simulink library "LIBRARY_SAD"  (R2025b)
settings: Solver=VariableStepAuto  StartTime=0.0  StopTime=10.0  RelTol=1e-3
values from neighbouring files (symbols this model uses):
  c = astroConstants(5)*1e3    [SCRIPT_SAD_DEMO.m]
  eps_E = deg2rad(astroConstants(63))    [SCRIPT_SAD_DEMO.m]
  F0 = 237    [SCRIPT_SAD_DEMO.m]
  F_e = 1358    [SCRIPT_SAD_DEMO.m]
  g = zeros(N, N+1)    [SCRIPT_SAD_DEMO.m]
  h = zeros(N, N+1)    [SCRIPT_SAD_DEMO.m]
  j_B = [0.01; 0.05; 0.01]    [SCRIPT_SAD_DEMO.m]
  JD0 = juliandate(startTime)    [SCRIPT_SAD_DEMO.m]
  mu = astroConstants(13)    [SCRIPT_SAD_DEMO.m]
  n = sqrt( (mu/ (a)^3))    [SCRIPT_SAD_DEMO.m]
  N = 13    [SCRIPT_SAD_DEMO.m]
  n_sun = 2*pi/T_sun    (= 1.99238499086e-07)    [SCRIPT_SAD_DEMO.m]
  r_sun = 1*AU    [SCRIPT_SAD_DEMO.m]
  Re = astroConstants(23)    [SCRIPT_SAD_DEMO.m]
  SRP = SRP_nom    [SCRIPT_SAD_DEMO.m]
  t0 = 0    [SCRIPT_SAD_DEMO.m]
  theta = 0    [SCRIPT_SAD_DEMO.m]
  w0 = w0_nom    [SCRIPT_SAD_DEMO.m]
  w_E = deg2rad(15.04)/3600    [SCRIPT_SAD_DEMO.m]
undefined symbols (not defined in the file or in its folder): g0_1, g1_1, h1_1, Ix, Iy, Iz, phi0, psi0, theta0
libraries: matrix_library x13, lIBRARY_SAD_SAD x12, $bdroot x5, LIBRARY_SAD_SAD x3, simulink x1
(part 1 of 2)
settings Model: Creator=fabio  LastModifiedBy=tomasfadista

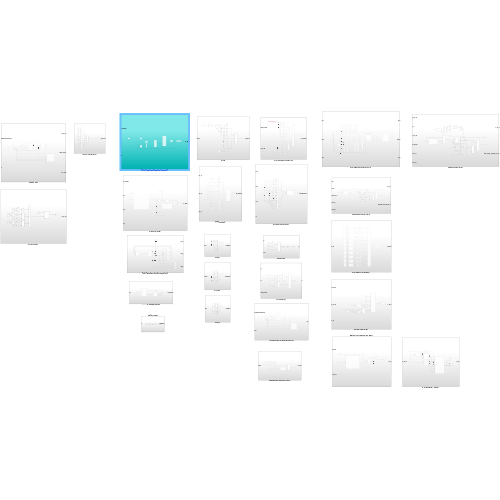
[thumbnail: Simulink's stored preview of the top-level diagram]
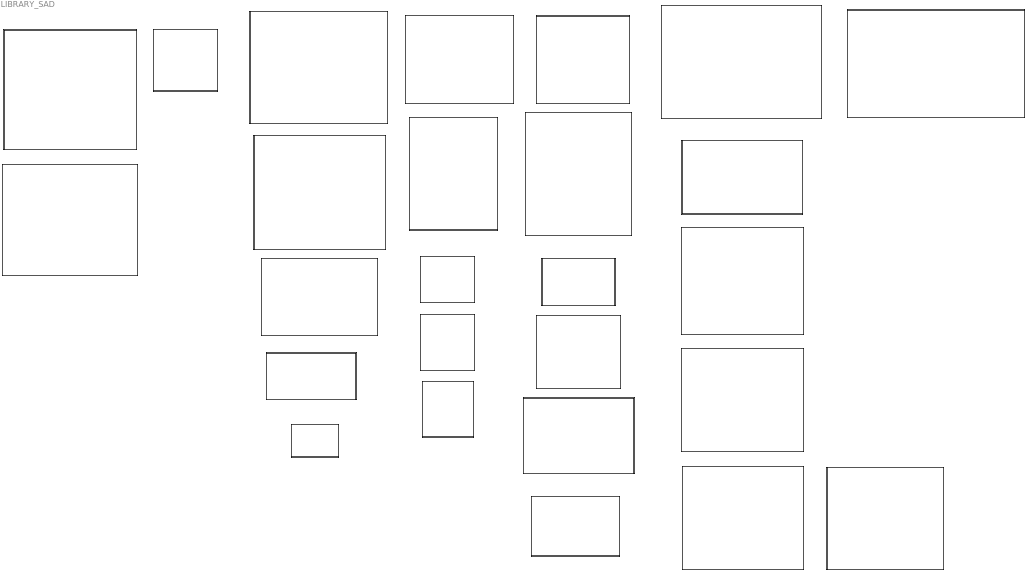
== system LIBRARY_SAD ==
  A1(theta) : Subsystem
  A2(psi) : Subsystem
  A3(phi) : Subsystem
  A_LVLH : Subsystem
  A_LVLH (elliptical,inclined orbit) : Subsystem
  B_N (IGRF Model - Order N) : Subsystem
  Conic Equation : Subsystem
  DCM Orthonormalisation : Subsystem
  DCM w matrix : Subsystem
  Earth Radiation Pressure : Subsystem
  Earth's Magnetic Dipole (unit vector) : Subsystem
  Earth-S/C Orbit : Subsystem
  Euler Angles Kinematics (seq. 312) : Subsystem
  "Euler Equations (scalar, torque-free)" : Subsystem
  Euler Equations Dynamics (vectorial) : Subsystem
  Gravity Gradient Torque : Subsystem
  I_matrix (principal axis) : Subsystem
  Kinematics (DCM) : Subsystem
  "Magnetic Torque (Simple Dipole Model) " : Subsystem
  Orbital Period : Subsystem
  Quaternion Omega matrix : Subsystem
  Solar Radiation Pressure Force : Subsystem
  Solar Radiation Torque (SRP) : Subsystem
  Sun-Earth Orbit : Subsystem
  Two-body Dynamics (keplerian elements) : Subsystem
  vector_norm : Subsystem

== system LIBRARY_SAD/A1(theta) ==
  theta : Inport
  Constant{,1,3..4} (4 alike) : Constant  Value=0
  Constant2 : Constant
  Cos : Trigonometry  Operator=cos
  Cos1 : Trigonometry  Operator=cos
  Gain : Gain  Gain=-1
  Sin : Trigonometry
  Sin1 : Trigonometry
  Vector Concatenate : Concatenate  NumInputs=3
  Vector Concatenate1 : Concatenate  NumInputs=3
  Vector Concatenate2 : Concatenate  NumInputs=3
  Vector Concatenate3 : Concatenate  NumInputs=3  Mode=Multidimensional array  ConcatenateDimension=2
  A1(theta) : Outport
  wires:
  Vector Concatenate3/1 -> A1(theta)/1
  Vector Concatenate2/1 -> Vector Concatenate3/1
  Vector Concatenate1/1 -> Vector Concatenate3/3
  Constant2/1 -> Vector Concatenate2/1
  Constant3/1 -> Vector Concatenate2/2
  Constant4/1 -> Vector Concatenate2/3
  Constant1/1 -> Vector Concatenate1/1
  Cos1/1 -> Vector Concatenate1/3
  Sin1/1 -> Vector Concatenate1/2
  Vector Concatenate/1 -> Vector Concatenate3/2
  Constant/1 -> Vector Concatenate/1
  Gain/1 -> Vector Concatenate/3
  Cos/1 -> Vector Concatenate/2
  Sin/1 -> Gain/1
  theta/1 -> Cos1/1, Sin1/1, Sin/1, Cos/1

== system LIBRARY_SAD/A2(psi) ==
  psi : Inport
  Constant{,1,3..4} (4 alike) : Constant  Value=0
  Constant2 : Constant
  Cos : Trigonometry  Operator=cos
  Cos1 : Trigonometry  Operator=cos
  Gain : Gain  Gain=-1
  Sin : Trigonometry
  Sin1 : Trigonometry
  Vector Concatenate : Concatenate  NumInputs=3
  Vector Concatenate1 : Concatenate  NumInputs=3
  Vector Concatenate2 : Concatenate  NumInputs=3
  Vector Concatenate3 : Concatenate  NumInputs=3  Mode=Multidimensional array  ConcatenateDimension=2
  A2(psi) : Outport
  wires:
  psi/1 -> Cos1/1, Sin1/1, Sin/1, Cos/1
  Vector Concatenate/1 -> Vector Concatenate3/2
  Vector Concatenate1/1 -> Vector Concatenate3/3
  Vector Concatenate2/1 -> Vector Concatenate3/1
  Vector Concatenate3/1 -> A2(psi)/1
  Cos/1 -> Vector Concatenate2/1
  Constant/1 -> Vector Concatenate2/2
  Sin/1 -> Vector Concatenate2/3
  Constant1/1 -> Vector Concatenate/1
  Constant2/1 -> Vector Concatenate/2
  Constant3/1 -> Vector Concatenate/3
  Sin1/1 -> Gain/1
  Constant4/1 -> Vector Concatenate1/2
  Cos1/1 -> Vector Concatenate1/3
  Gain/1 -> Vector Concatenate1/1

== system LIBRARY_SAD/A3(phi) ==
  phi : Inport
  Constant{,1..3} (4 alike) : Constant  Value=0
  Constant4 : Constant
  Cos : Trigonometry  Operator=cos
  Cos1 : Trigonometry  Operator=cos
  Gain : Gain  Gain=-1
  Sin : Trigonometry
  Sin1 : Trigonometry
  Vector Concatenate : Concatenate  NumInputs=3
  Vector Concatenate1 : Concatenate  NumInputs=3
  Vector Concatenate2 : Concatenate  NumInputs=3
  Vector Concatenate3 : Concatenate  NumInputs=3  Mode=Multidimensional array  ConcatenateDimension=2
  A3(phi) : Outport
  wires:
  phi/1 -> Sin1/1, Cos/1, Sin/1, Cos1/1
  Sin/1 -> Gain/1
  Cos/1 -> Vector Concatenate/1
  Gain/1 -> Vector Concatenate/2
  Constant/1 -> Vector Concatenate/3
  Vector Concatenate/1 -> Vector Concatenate3/1
  Sin1/1 -> Vector Concatenate1/1
  Cos1/1 -> Vector Concatenate1/2
  Constant1/1 -> Vector Concatenate1/3
  Constant4/1 -> Vector Concatenate2/3
  Constant3/1 -> Vector Concatenate2/2
  Constant2/1 -> Vector Concatenate2/1
  Vector Concatenate1/1 -> Vector Concatenate3/2
  Vector Concatenate2/1 -> Vector Concatenate3/3
  Vector Concatenate3/1 -> A3(phi)/1

== system LIBRARY_SAD/A_LVLH ==
  Time : Inport
  Constant : Constant  Value=0
  Constant1 : Constant
  Cos : Trigonometry  Operator=cos
  Gain1 : Gain  Gain=n
  Gain2 : Gain  Gain=-1
  Sin : Trigonometry
  Vector Concatenate : Concatenate  NumInputs=3
  Vector Concatenate1 : Concatenate  NumInputs=3
  Vector Concatenate2 : Concatenate  NumInputs=3
  Vector Concatenate3 : Concatenate  NumInputs=3  Mode=Multidimensional array  ConcatenateDimension=2
  A_LVLH : Outport
  wires:
  Constant/1 -> Vector Concatenate2/2, Vector Concatenate2/1, Vector Concatenate1/3, Vector Concatenate/3
  Gain2/1 -> Vector Concatenate/2
  Cos/1 -> Vector Concatenate1/2, Vector Concatenate/1
  Gain1/1 -> Sin/1, Cos/1
  Sin/1 -> Vector Concatenate1/1, Gain2/1
  Vector Concatenate1/1 -> Vector Concatenate3/2
  Vector Concatenate3/1 -> A_LVLH/1
  Vector Concatenate2/1 -> Vector Concatenate3/3
  Vector Concatenate/1 -> Vector Concatenate3/1
  Time/1 -> Gain1/1
  Constant1/1 -> Vector Concatenate2/3

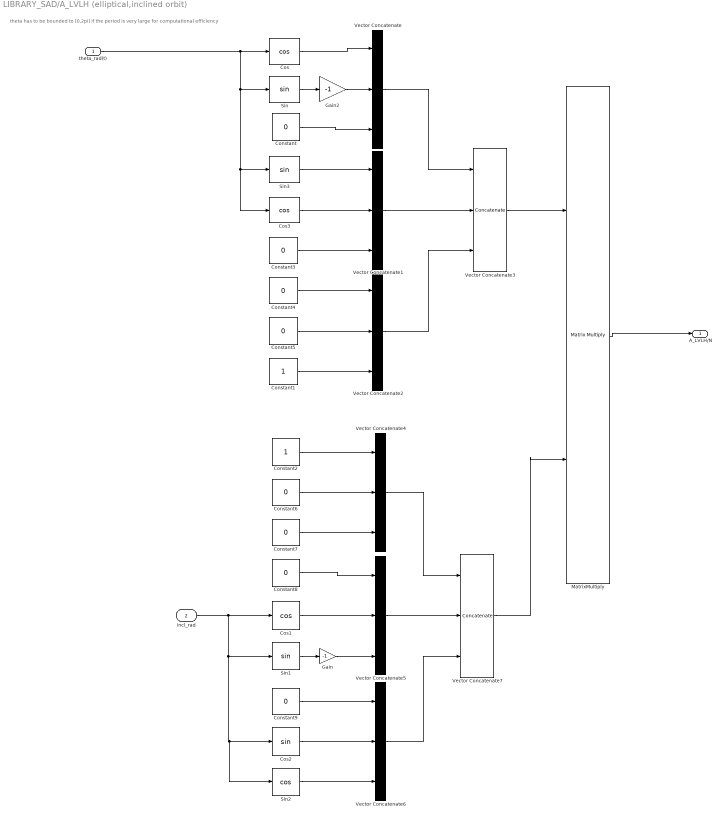
== system LIBRARY_SAD/A_LVLH (elliptical,inclined orbit) ==
  note: theta has to be bounded to [0,2pi] if the period is very large for computational efficiency
  theta_rad(t) : Inport
  incl_rad : Inport  Port=2
  Constant{,3..9} (8 alike) : Constant  Value=0
  Constant1 : Constant
  Constant2 : Constant
  Cos : Trigonometry  Operator=cos
  Cos1 : Trigonometry  Operator=cos
  Cos2 : Trigonometry
  Cos3 : Trigonometry  Operator=cos
  Gain : Gain  Gain=-1
  Gain2 : Gain  Gain=-1
  MatrixMultiply : Product  Multiplication=Matrix(*)
  Sin : Trigonometry
  Sin1 : Trigonometry
  Sin2 : Trigonometry  Operator=cos
  Sin3 : Trigonometry
  Vector Concatenate{,1..2,4..6} (6 alike) : Concatenate  NumInputs=3
  Vector Concatenate3 : Concatenate  NumInputs=3  Mode=Multidimensional array  ConcatenateDimension=2
  Vector Concatenate7 : Concatenate  NumInputs=3  Mode=Multidimensional array  ConcatenateDimension=2
  A_LVLH/N : Outport
  wires:
  Constant/1 -> Vector Concatenate/3
  Gain2/1 -> Vector Concatenate/2
  Cos/1 -> Vector Concatenate/1
  theta_rad(t)/1 -> Cos3/1, Sin3/1, Sin/1, Cos/1
  Sin/1 -> Gain2/1
  Vector Concatenate1/1 -> Vector Concatenate3/2
  Vector Concatenate3/1 -> MatrixMultiply/1
  Vector Concatenate2/1 -> Vector Concatenate3/3
  Vector Concatenate/1 -> Vector Concatenate3/1
  Constant1/1 -> Vector Concatenate2/3
  MatrixMultiply/1 -> A_LVLH/N/1
  Constant2/1 -> Vector Concatenate4/1
  incl_rad/1 -> Sin2/1, Cos2/1, Sin1/1, Cos1/1
  Cos1/1 -> Vector Concatenate5/2
  Sin1/1 -> Gain/1
  Gain/1 -> Vector Concatenate5/3
  Cos2/1 -> Vector Concatenate6/2
  Sin2/1 -> Vector Concatenate6/3
  Vector Concatenate5/1 -> Vector Concatenate7/2
  Vector Concatenate4/1 -> Vector Concatenate7/1
  Vector Concatenate6/1 -> Vector Concatenate7/3
  Vector Concatenate7/1 -> MatrixMultiply/2
  Sin3/1 -> Vector Concatenate1/1
  Cos3/1 -> Vector Concatenate1/2
  Constant3/1 -> Vector Concatenate1/3
  Constant4/1 -> Vector Concatenate2/1
  Constant5/1 -> Vector Concatenate2/2
  Constant6/1 -> Vector Concatenate4/2
  Constant7/1 -> Vector Concatenate4/3
  Constant8/1 -> Vector Concatenate5/1
  Constant9/1 -> Vector Concatenate6/1

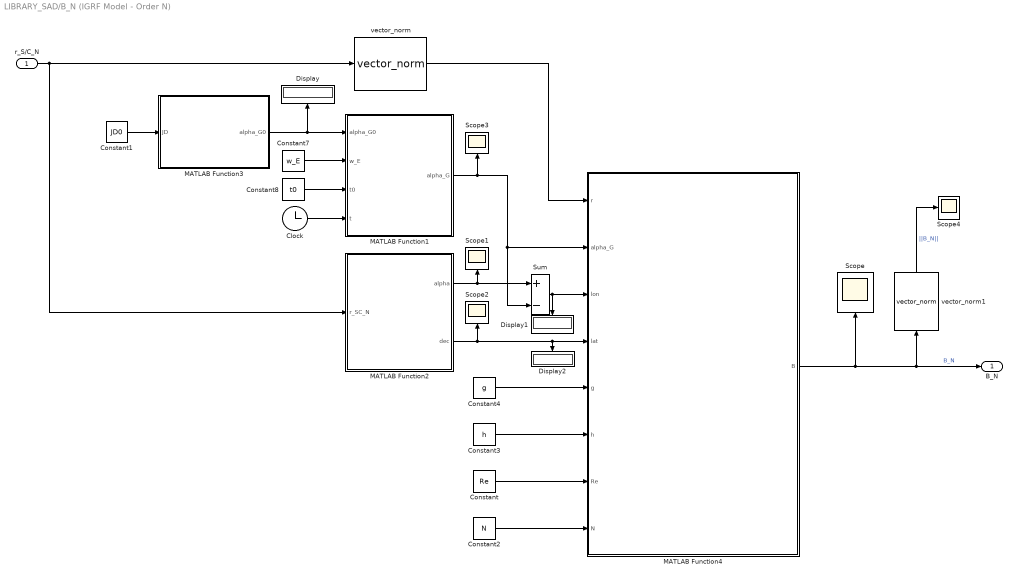
== system LIBRARY_SAD/B_N (IGRF Model - Order N) ==
  r_S/C_N : Inport
  Clock : Clock
  Constant : Constant  Value=Re
  Constant1 : Constant  Value=JD0
  Constant2 : Constant  Value=N
  Constant3 : Constant  Value=h
  Constant4 : Constant  Value=g
  Constant7 : Constant  Value=w_E
  Constant8 : Constant  Value=t0
  Display : Display
  Display1 : Display
  Display2 : Display
  MATLAB Function1 : MATLAB Function  TreatAsAtomicUnit=on
  MATLAB Function2 : MATLAB Function  TreatAsAtomicUnit=on
  MATLAB Function3 : MATLAB Function  TreatAsAtomicUnit=on
  MATLAB Function4 : MATLAB Function  TreatAsAtomicUnit=on
  Scope{,1..4} (5 alike) : Scope
      Scope settings: ActiveDisplayYMinimum=-1.512041376614329E-5  ActiveDisplayYMaximum=2.8400469726666671E-5  DataLoggingVariableName=ScopeData27
      Scope1 settings: ActiveDisplayYMinimum=-1  ActiveDisplayYMaximum=1  DataLoggingVariableName=ScopeData28
      Scope2 settings: ActiveDisplayYMinimum=-1  ActiveDisplayYMaximum=1  DataLoggingVariableName=ScopeData29
      Scope3 settings: ActiveDisplayYMinimum=-1  ActiveDisplayYMaximum=1  DataLoggingVariableName=ScopeData30
      Scope4 settings: ActiveDisplayYMinimum=-1  ActiveDisplayYMaximum=1  DataLoggingVariableName=ScopeData32
  Sum : Sum  Inputs=+-
  vector_norm : $bdroot/vector_norm  SystemSampleTime=-1  VariantActivationTime=update diagram  EmptyChoice=off  PassThrough=off  PassThroughVariantControl=(default)  EmptyChoiceVariantControl=(default)  AllowFlexibleInterface=on  Latency=0  AutoFrameSizeCalculation=off
  vector_norm1 : $bdroot/vector_norm  SystemSampleTime=-1  VariantActivationTime=update diagram  EmptyChoice=off  PassThrough=off  PassThroughVariantControl=(default)  EmptyChoiceVariantControl=(default)  AllowFlexibleInterface=on  Latency=0  AutoFrameSizeCalculation=off
  B_N : Outport
  wires:
  Constant1/1 -> MATLAB Function3/1(JD)
  MATLAB Function2/1(alpha) -> Sum/1, Scope1/1
  Sum/1 -> Display1/1, MATLAB Function4/3(lon)
  MATLAB Function2/2(dec) -> Display2/1, MATLAB Function4/4(lat), Scope2/1
  MATLAB Function1/1(alpha_G) -> Scope3/1, Sum/2, MATLAB Function4/2(alpha_G)
  Clock/1 -> MATLAB Function1/4(t)
  Constant8/1 -> MATLAB Function1/3(t0)
  Constant7/1 -> MATLAB Function1/2(w_E)
  vector_norm1/1 -> Scope4/1  "||B_N||"
  MATLAB Function4/1(B) -> Scope/1, vector_norm1/1, B_N/1  "B_N"
  Constant4/1 -> MATLAB Function4/5(g)
  Constant3/1 -> MATLAB Function4/6(h)
  Constant2/1 -> MATLAB Function4/8(N)
  MATLAB Function3/1(alpha_G0) -> Display/1, MATLAB Function1/1(alpha_G0)
  Constant/1 -> MATLAB Function4/7(Re)
  vector_norm/1 -> MATLAB Function4/1(r)
  r_S/C_N/1 -> vector_norm/1, MATLAB Function2/1(r_SC_N)

== system LIBRARY_SAD/Conic Equation ==
  a : Inport
  e : Inport  Port=2
  theta_rad(t) : Inport  Port=3
  Constant : Constant  Value=2
  Constant1 : Constant
  Constant2 : Constant
  Cos : Trigonometry  Operator=cos
  Divide : Product  Inputs=*/
  Power : Math  Operator=pow
  Product : Product
  Product1 : Product
  Sum : Sum  Inputs=+-
  Sum1 : Sum  Inputs=+-
  r : Outport
  wires:
  a/1 -> Product/1
  e/1 -> Product1/1, Power/1
  Constant/1 -> Power/2
  Power/1 -> Sum/2
  Constant1/1 -> Sum/1
  Sum/1 -> Product/2
  Product/1 -> Divide/1
  Divide/1 -> r/1
  Constant2/1 -> Sum1/1
  theta_rad(t)/1 -> Cos/1
  Cos/1 -> Product1/2
  Product1/1 -> Sum1/2
  Sum1/1 -> Divide/2

== system LIBRARY_SAD/DCM Orthonormalisation ==
  A : Inport
  Gain4 : Gain  Gain=3/2
  Gain5 : Gain  Gain=1/2
  Product1 : Product  Inputs=3  Multiplication=Matrix(*)
  Sum : Sum  Inputs=+-
  Transpose : Math  Operator=transpose
  A_ortho : Outport
  wires:
  Gain4/1 -> Sum/1
  Transpose/1 -> Product1/2
  Gain5/1 -> Sum/2
  Product1/1 -> Gain5/1
  A/1 -> Gain4/1, Product1/1, Transpose/1, Product1/3
  Sum/1 -> A_ortho/1

== system LIBRARY_SAD/DCM w matrix ==
  w_x : Inport
  w_y : Inport  Port=2
  w_z : Inport  Port=3
  Constant : Constant  Value=0
  Constant1 : Constant  Value=0
  Constant2 : Constant  Value=0
  Gain : Gain  Gain=-1
  Gain1 : Gain  Gain=-1
  Gain2 : Gain  Gain=-1
  Vector Concatenate : Concatenate  NumInputs=3  Mode=Multidimensional array
  Vector Concatenate1 : Concatenate  NumInputs=3  Mode=Multidimensional array
  Vector Concatenate2 : Concatenate  NumInputs=3  Mode=Multidimensional array
  Vector Concatenate3 : Concatenate  NumInputs=3  Mode=Multidimensional array  ConcatenateDimension=2
  w_matrix : Outport
  wires:
  Gain/1 -> Vector Concatenate/3
  w_z/1 -> Gain1/1, Vector Concatenate/2
  Constant2/1 -> Vector Concatenate2/3
  Gain2/1 -> Vector Concatenate2/2
  w_x/1 -> Vector Concatenate1/3, Gain2/1
  Vector Concatenate/1 -> Vector Concatenate3/1
  Constant1/1 -> Vector Concatenate1/2
  Vector Concatenate1/1 -> Vector Concatenate3/2
  w_y/1 -> Gain/1, Vector Concatenate2/1
  Gain1/1 -> Vector Concatenate1/1
  Constant/1 -> Vector Concatenate/1
  Vector Concatenate2/1 -> Vector Concatenate3/3
  Vector Concatenate3/1 -> w_matrix/1  "w_matrix"

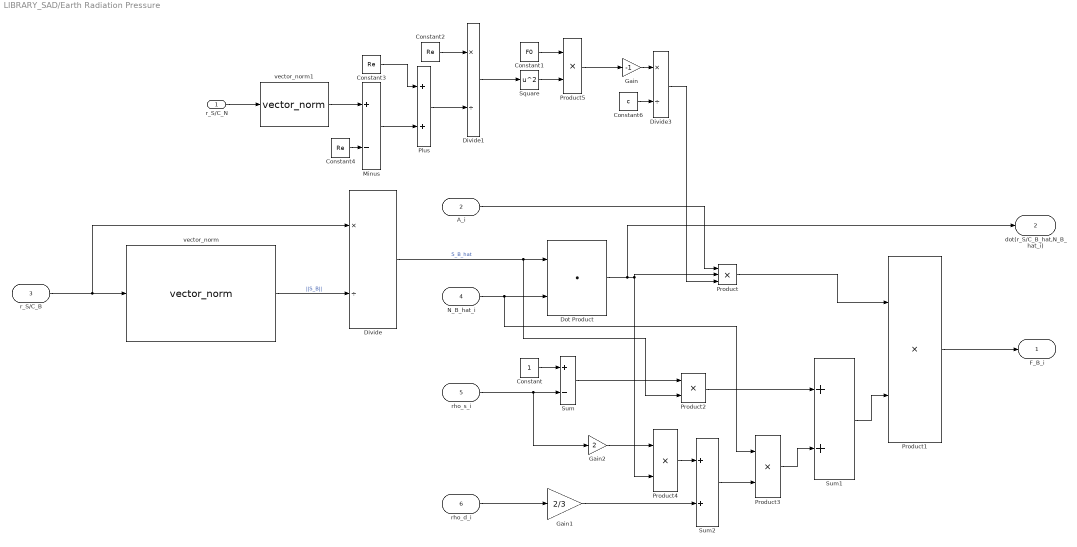
== system LIBRARY_SAD/Earth Radiation Pressure ==
  r_S/C_N : Inport
  A_i : Inport  Port=2
  r_S/C_B : Inport  Port=3
  N_B_hat_i : Inport  Port=4
  rho_s_i : Inport  Port=5
  rho_d_i : Inport  Port=6
  Constant : Constant
  Constant1 : Constant  Value=F0
  Constant2 : Constant  Value=Re
  Constant3 : Constant  Value=Re
  Constant4 : Constant  Value=Re
  Constant6 : Constant  Value=c
  Divide : Product  Inputs=*/
  Divide1 : Product  Inputs=*/
  Divide3 : Product  Inputs=*/
  Dot Product : DotProduct  OutDataTypeStr=Inherit: Inherit via internal rule
  Gain : Gain  Gain=-1
  Gain1 : Gain  Gain=2/3
  Gain2 : Gain  Gain=2
  Minus : Sum  Inputs=+-
  Plus : Sum
  Product : Product  Inputs=3
  Product{1..5} (5 alike) : Product
  Square : Math  Operator=square
  Sum : Sum  Inputs=+-
  Sum1 : Sum
  Sum2 : Sum
  vector_norm : $bdroot/vector_norm  SystemSampleTime=-1  VariantActivationTime=update diagram  EmptyChoice=off  PassThrough=off  PassThroughVariantControl=(default)  EmptyChoiceVariantControl=(default)  AllowFlexibleInterface=on  Latency=0  AutoFrameSizeCalculation=off
  vector_norm1 : $bdroot/vector_norm  SystemSampleTime=-1  VariantActivationTime=update diagram  EmptyChoice=off  PassThrough=off  PassThroughVariantControl=(default)  EmptyChoiceVariantControl=(default)  AllowFlexibleInterface=on  Latency=0  AutoFrameSizeCalculation=off
  F_B_i : Outport
  dot(r_S/C_B_hat,N_B_hat_i) : Outport  Port=2
  wires:
  Sum1/1 -> Product1/2
  A_i/1 -> Product/1
  N_B_hat_i/1 -> Product3/1, Dot Product/2
  vector_norm/1 -> Divide/2  "||S_B||"
  Product4/1 -> Sum2/1
  Product2/1 -> Sum1/1
  Product1/1 -> F_B_i/1
  Gain1/1 -> Sum2/2
  Divide/1 -> Product2/2, Dot Product/1  "S_B_hat"
  Product3/1 -> Sum1/2
  Product/1 -> Product1/1
  rho_d_i/1 -> Gain1/1
  Constant/1 -> Sum/1
  Sum/1 -> Product2/1
  Sum2/1 -> Product3/2
  r_S/C_B/1 -> vector_norm/1, Divide/1
  rho_s_i/1 -> Gain2/1, Sum/2
  Gain2/1 -> Product4/1
  Dot Product/1 -> dot(r_S/C_B_hat,N_B_hat_i)/1, Product/2, Product4/2
  Product5/1 -> Gain/1
  Constant2/1 -> Divide1/1
  Plus/1 -> Divide1/2
  Constant3/1 -> Plus/1
  Minus/1 -> Plus/2
  Divide1/1 -> Square/1
  Square/1 -> Product5/2
  Constant1/1 -> Product5/1
  Gain/1 -> Divide3/1
  Constant6/1 -> Divide3/2
  Divide3/1 -> Product/3
  r_S/C_N/1 -> vector_norm1/1
  Constant4/1 -> Minus/2
  vector_norm1/1 -> Minus/1

== system LIBRARY_SAD/Earth's Magnetic Dipole (unit vector) ==
  Time : Inport
  Constant : Constant  Value=11.5
  Constant2 : Constant  Value=11.5
  Cos : Trigonometry  Operator=cos
  Cos1 : Trigonometry
  Divide : Product  Inputs=*/
  Gain : Gain  Gain=w_E
  Gain1 : Gain  Gain=pi/180
  Gain2 : Gain  Gain=w_E
  Gain4 : Gain  Gain=pi/180
  Product : Product
  Product1 : Product
  Sin : Trigonometry
  Sin2 : Trigonometry  Operator=cos
  Vector Concatenate : Concatenate  NumInputs=3
  vector_norm : LIBRARY_SAD_SAD/vector_norm  SystemSampleTime=-1  SSRTWFcnClass=[]  VariantActivationTime=update diagram  EmptyChoice=off  PassThrough=off  PassThroughVariantControl=(default)  EmptyChoiceVariantControl=(default)  AllowFlexibleInterface=on  Latency=0  AutoFrameSizeCalculation=off
  m_hat : Outport
  wires:
  Gain/1 -> Cos/1
  Cos/1 -> Product/1
  Sin/1 -> Product/2, Product1/2
  Constant/1 -> Gain1/1
  Gain1/1 -> Sin/1
  Product/1 -> Vector Concatenate/1
  Product1/1 -> Vector Concatenate/2
  Cos1/1 -> Product1/1
  Gain2/1 -> Cos1/1
  Time/1 -> Gain2/1, Gain/1
  Constant2/1 -> Gain4/1
  Gain4/1 -> Sin2/1
  Sin2/1 -> Vector Concatenate/3
  Vector Concatenate/1 -> vector_norm/1, Divide/1  "m"
  Divide/1 -> m_hat/1
  vector_norm/1 -> Divide/2

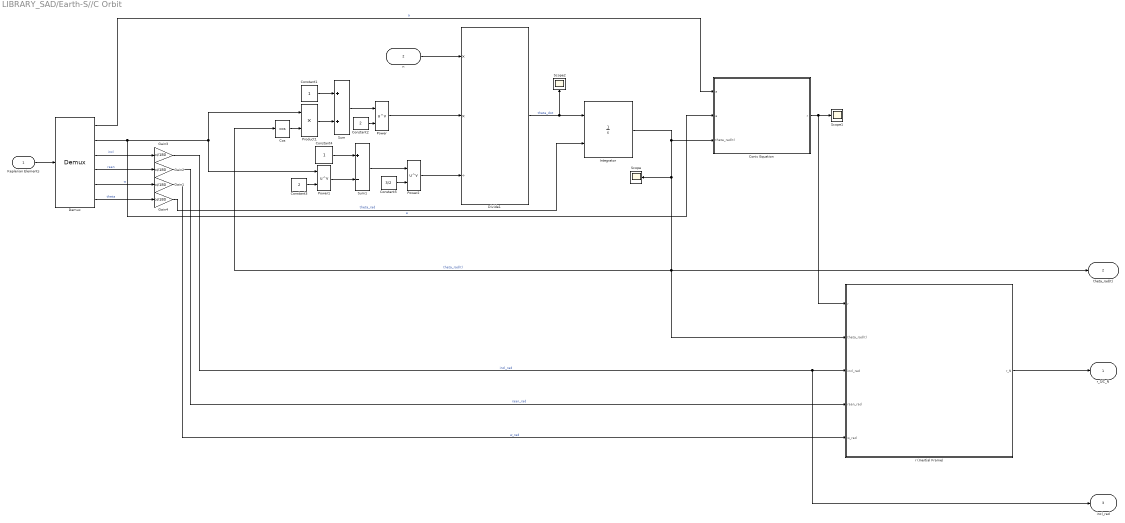
== system LIBRARY_SAD/Earth-S//C Orbit ==
  Keplerian Elements : Inport
  n : Inport  Port=2
  Conic Equation : Subsystem
  Constant1 : Constant
  Constant2 : Constant  Value=2
  Constant3 : Constant  Value=2
  Constant4 : Constant
  Constant5 : Constant  Value=3/2
  Cos : Trigonometry  Operator=cos
  Demux : Demux  Outputs=6
      settings: DisplayOption=none
  Divide1 : Product  Inputs=**/
  Gain{1..4} (4 alike) : Gain  Gain=pi/180
  Integrator : Integrator  InitialConditionSource=external  InitialCondition=theta  WrapState=on  WrappedStateUpperValue=2*pi  WrappedStateLowerValue=0
  Power : Math  Operator=pow
  Power1 : Math  Operator=pow
  Power2 : Math  Operator=pow
  Product1 : Product
  Scope : Scope
      settings: ActiveDisplayYMinimum=-0.785387370168924  ActiveDisplayYMaximum=7.0684863315203179  DataLoggingVariableName=ScopeData22
  Scope1 : Scope
      settings: ActiveDisplayYMinimum=6287.5500000061184  ActiveDisplayYMaximum=10412.44999994494  DataLoggingVariableName=ScopeData23
  Scope2 : Scope
      settings: ActiveDisplayYMinimum=0.00072744506449318766  ActiveDisplayYMaximum=0.00092744506449318775  DataLoggingVariableName=ScopeData24
  Sum : Sum
  Sum1 : Sum  Inputs=+-
  r (Inertial Frame) : Subsystem
  r_S/C_N : Outport
  theta_rad(t) : Outport  Port=2
  incl_rad : Outport  Port=3
  wires:
  Keplerian Elements/1 -> Demux/1
  Demux/1 -> Conic Equation/1(a)  "a"
  Demux/2 -> Conic Equation/2(e), Product1/1, Power1/1  "e"
  Demux/3 -> Gain3/1  "incl"
  Demux/4 -> Gain2/1  "raan"
  Demux/5 -> Gain1/1  "w"
  Demux/6 -> Gain4/1  "theta"
  Constant1/1 -> Sum/1
  Cos/1 -> Product1/2
  Product1/1 -> Sum/2
  Sum/1 -> Power/1
  Constant2/1 -> Power/2
  Power/1 -> Divide1/2
  Constant3/1 -> Power1/2
  Power1/1 -> Sum1/2
  Constant4/1 -> Sum1/1
  Constant5/1 -> Power2/2
  Sum1/1 -> Power2/1
  Power2/1 -> Divide1/3
  Divide1/1 -> Scope2/1, Integrator/1  "theta_dot"
  Integrator/1 -> Scope/1, Cos/1, r (Inertial Frame)/2(theta_rad(t)), theta_rad(t)/1, Conic Equation/3(theta_rad(t))  "theta_rad(t)"
  Conic Equation/1(r) -> r (Inertial Frame)/1(r), Scope1/1
  Gain3/1 -> incl_rad/1, r (Inertial Frame)/3(incl_rad)  "incl_rad"
  Gain2/1 -> r (Inertial Frame)/4(raan_rad)  "raan_rad"
  Gain1/1 -> r (Inertial Frame)/5(w_rad)  "w_rad"
  r (Inertial Frame)/1(r_N) -> r_S/C_N/1
  n/1 -> Divide1/1
  Gain4/1 -> Integrator/2  "theta_rad"

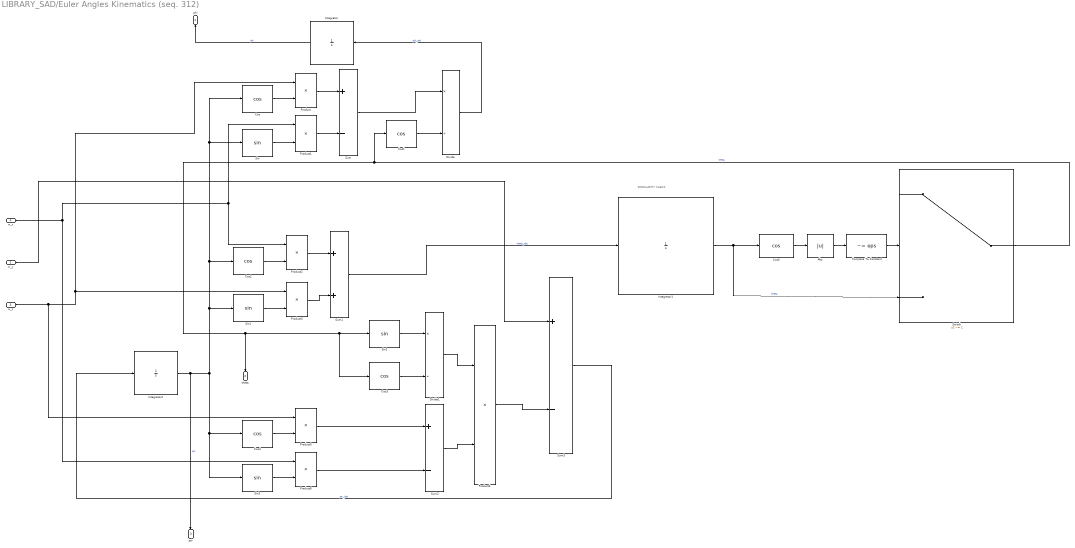
== system LIBRARY_SAD/Euler Angles Kinematics (seq. 312) ==
  note: SINGULARITY CHECK
  w_x : Inport
  w_y : Inport  Port=2
  w_z : Inport  Port=3
  Abs : Abs  SaturateOnIntegerOverflow=off
  Compare To Constant : simulink/Logic and Bit Operations/Compare To Constant  relop=~=  const=eps  OutDataTypeStr=boolean
  Cos{,1..5} (6 alike) : Trigonometry  Operator=cos
  Divide : Product  Inputs=*/
  Divide1 : Product  Inputs=*/
  Integrator : Integrator  InitialCondition=phi0
  Integrator1 : Integrator  InitialCondition=theta0  UpperSaturationLimit=+pi/2  LowerSaturationLimit=-pi/2
  Integrator2 : Integrator  InitialCondition=psi0
  Product{,1..6} (7 alike) : Product
  Sin{,1..3} (4 alike) : Trigonometry
  Sum : Sum  Inputs=+-
  Sum1 : Sum
  Sum2 : Sum  Inputs=+-
  Sum3 : Sum  Inputs=+-
  Switch : Switch  Threshold=1  SaturateOnIntegerOverflow=off  InputSameDT=off
  phi : Outport
  theta : Outport  Port=2
  psi : Outport  Port=3
  wires:
  w_z/1 -> Product/1, Product3/1, Product5/1
  Product/1 -> Sum/1
  Divide1/1 -> Product4/1
  Sum/1 -> Divide/1
  Cos2/1 -> Product2/2
  Divide/1 -> Integrator/1  "phi_dot"
  Sin/1 -> Product1/2
  Sum1/1 -> Integrator1/1  "theta_dot"
  Product6/1 -> Sum2/2
  Cos4/1 -> Product5/2
  w_x/1 -> Product1/1, Product2/1, Product6/1
  Integrator2/1 -> Sin/1, Cos/1, Cos2/1, Sin1/1, Cos4/1, Sin3/1, psi/1  "psi"
  Cos/1 -> Product/2
  Sin1/1 -> Product3/2
  Product2/1 -> Sum1/1
  Product1/1 -> Sum/2
  Cos3/1 -> Divide1/2
  Sin3/1 -> Product6/2
  Product4/1 -> Sum3/2
  Integrator/1 -> phi/1  "phi"
  Sin2/1 -> Divide1/1
  Integrator1/1 -> Cos5/1, Switch/3  "theta"
  Cos1/1 -> Divide/2
  Product3/1 -> Sum1/2
  Product5/1 -> Sum2/1
  Sum3/1 -> Integrator2/1  "psi_dot"
  Sum2/1 -> Product4/2
  w_y/1 -> Sum3/1
  Cos5/1 -> Abs/1
  Compare To Constant/1 -> Switch/2
  Abs/1 -> Compare To Constant/1
  Switch/1 -> Cos1/1, Cos3/1, Sin2/1, theta/1  "theta"

== system LIBRARY_SAD/Euler Equations (scalar, torque-free) ==
  Demux : Demux  Outputs=3
      settings: DisplayOption=none
  Integrator : Integrator  InitialCondition=w0
  Mux : Mux  Inputs=3
  Scope : Scope  NumInputPorts=3
      settings: ActiveDisplayYMinimum=-1  ActiveDisplayYMaximum=1
  To Workspace : ToWorkspace  VariableName=w_x  SampleTime=-1
  To Workspace1 : ToWorkspace  VariableName=w_y  SampleTime=-1
  To Workspace2 : ToWorkspace  VariableName=w_z  SampleTime=-1
  w_x_dot : Subsystem
  w_y_dot : Subsystem
  w_z_dot : Subsystem
  w_x : Outport
  w_y : Outport  Port=2
  w_z : Outport  Port=3
  wires:
  w_x_dot/1(w_x_dot) -> Mux/1
  Demux/2 -> Scope/2, w_x_dot/1(w_y), w_z_dot/2(w_y), To Workspace1/1, w_y/1  "w_y"
  Demux/3 -> To Workspace2/1, Scope/3, w_y_dot/2(w_z), w_x_dot/2(w_z), w_z/1  "w_z"
  w_y_dot/1(w_y_dot) -> Mux/2
  Demux/1 -> To Workspace/1, w_x/1, Scope/1, w_y_dot/1(w_x), w_z_dot/1(w_x)  "w_x"
  Mux/1 -> Integrator/1  "w_dot"
  w_z_dot/1(w_z_dot) -> Mux/3
  Integrator/1 -> Demux/1  "w"

== system LIBRARY_SAD/Euler Equations Dynamics (vectorial) ==
  I_matrix : Inport
  T : Inport  Port=2
  Cross Product : matrix_library/Cross Product
  Integrator : Integrator  InitialCondition=w0
  Matrix Divide : Product  Inputs=/  Multiplication=Matrix(*)
  MatrixMultiply : Product  Multiplication=Matrix(*)
  Product : Product  Multiplication=Matrix(*)
  Sum : Sum  Inputs=+-
  w_B : Outport
  wires:
  Sum/1 -> Product/2
  MatrixMultiply/1 -> Cross Product/2
  Cross Product/1 -> Sum/2
  T/1 -> Sum/1
  Product/1 -> Integrator/1  "w_dot"
  Integrator/1 -> w_B/1, MatrixMultiply/2, Cross Product/1  "w"
  I_matrix/1 -> Matrix Divide/1, MatrixMultiply/1  "I_matrix"
  Matrix Divide/1 -> Product/1  "(I_matrix)^-1"

== system LIBRARY_SAD/Gravity Gradient Torque ==
  I_matrix : Inport
  r_S/C_B : Inport  Port=2
  c_B : Inport  Port=3
  Constant : Constant  Value=3
  Constant1 : Constant  Value=mu
  Constant4 : Constant  Value=3
  Cross Product : matrix_library/Cross Product
  Divide : Product  Inputs=**/*
  MatrixMultiply : Product  Multiplication=Matrix(*)
  Power : Math  Operator=pow
  vector_norm : LIBRARY_SAD_SAD/vector_norm  SystemSampleTime=-1  SSRTWFcnClass=[]  VariantActivationTime=update diagram  EmptyChoice=off  PassThrough=off  PassThroughVariantControl=(default)  EmptyChoiceVariantControl=(default)  AllowFlexibleInterface=on  Latency=0  AutoFrameSizeCalculation=off
  T_GG : Outport
  wires:
  r_S/C_B/1 -> vector_norm/1
  Constant4/1 -> Power/2
  Constant/1 -> Divide/1
  Constant1/1 -> Divide/2
  Power/1 -> Divide/3
  I_matrix/1 -> MatrixMultiply/1
  c_B/1 -> MatrixMultiply/2, Cross Product/1
  MatrixMultiply/1 -> Cross Product/2
  Cross Product/1 -> Divide/4
  Divide/1 -> T_GG/1
  vector_norm/1 -> Power/1

== system LIBRARY_SAD/I_matrix (principal axis) ==
  Constant : Constant  Value=Ix
  Constant{1..3,5..7} (6 alike) : Constant  Value=0
  Constant4 : Constant  Value=Iy
  Constant8 : Constant  Value=Iz
  Vector Concatenate : Concatenate  NumInputs=3
  Vector Concatenate1 : Concatenate  NumInputs=3
  Vector Concatenate2 : Concatenate  NumInputs=3
  Vector Concatenate3 : Concatenate  NumInputs=3  Mode=Multidimensional array  ConcatenateDimension=2
  I_matrix : Outport
  wires:
  Vector Concatenate3/1 -> I_matrix/1
  Constant/1 -> Vector Concatenate/1
  Constant1/1 -> Vector Concatenate/2
  Constant2/1 -> Vector Concatenate/3
  Vector Concatenate/1 -> Vector Concatenate3/1
  Constant3/1 -> Vector Concatenate1/1
  Constant4/1 -> Vector Concatenate1/2
  Constant5/1 -> Vector Concatenate1/3
  Constant6/1 -> Vector Concatenate2/1
  Constant7/1 -> Vector Concatenate2/2
  Constant8/1 -> Vector Concatenate2/3
  Vector Concatenate1/1 -> Vector Concatenate3/2
  Vector Concatenate2/1 -> Vector Concatenate3/3

== system LIBRARY_SAD/Kinematics (DCM) ==
  A_LVLH/N : Inport
  w_x : Inport  Port=2
  w_y : Inport  Port=3
  w_z : Inport  Port=4
  DCM Orthonormalisation : LIBRARY_SAD_SAD/DCM Orthonormalisation  SystemSampleTime=-1  SSRTWFcnClass=[]  VariantActivationTime=update diagram  EmptyChoice=off  PassThrough=off  PassThroughVariantControl=(default)  EmptyChoiceVariantControl=(default)  AllowFlexibleInterface=on  Latency=0  AutoFrameSizeCalculation=off
  DCM w matrix : lIBRARY_SAD_SAD/DCM w matrix  SystemSampleTime=-1  SSRTWFcnClass=[]  VariantActivationTime=update diagram  EmptyChoice=off  PassThrough=off  PassThroughVariantControl=(default)  EmptyChoiceVariantControl=(default)  AllowFlexibleInterface=on  Latency=0  AutoFrameSizeCalculation=off
  Gain : Gain  Gain=-1
  Integrator : Integrator  InitialConditionSource=external
  Product : Product  Multiplication=Matrix(*)
  To Workspace : ToWorkspace  VariableName=A_B_N  SampleTime=-1
  To Workspace1 : ToWorkspace  VariableName=A_B_N_ortho  SampleTime=-1
  A_B/N : Outport
  wires:
  A_LVLH/N/1 -> Integrator/2
  w_y/1 -> DCM w matrix/2
  w_z/1 -> DCM w matrix/3
  Integrator/1 -> To Workspace/1, DCM Orthonormalisation/1  "A_B/N"
  Product/1 -> Integrator/1  "A_dot"
  DCM w matrix/1 -> Gain/1
  w_x/1 -> DCM w matrix/1
  Gain/1 -> Product/1
  DCM Orthonormalisation/1 -> To Workspace1/1, A_B/N/1, Product/2  "A_B/N"

== system LIBRARY_SAD/Magnetic Torque (Simple Dipole Model)  ==
  A_B/N : Inport
  r_S/C_N : Inport  Port=2
  B_N (Simple Dipole Model) : Subsystem
  Constant : Constant  Value=j_B
  Cross Product : matrix_library/Cross Product
  MatrixMultiply : Product  Multiplication=Matrix(*)
  Scope : Scope
      settings: ActiveDisplayYMinimum=-1  ActiveDisplayYMaximum=1  DataLoggingVariableName=ScopeData5
  T_M : Outport
  wires:
  r_S/C_N/1 -> B_N (Simple Dipole Model)/1(r_S/C_N)
  B_N (Simple Dipole Model)/1(B_N) -> MatrixMultiply/2
  A_B/N/1 -> MatrixMultiply/1
  MatrixMultiply/1 -> Scope/1, Cross Product/2  "B_B"
  Constant/1 -> Cross Product/1
  Cross Product/1 -> T_M/1

== system LIBRARY_SAD/Orbital Period ==
  a : Inport
  mu : Inport  Port=2
  Constant : Constant  Value=3
  Divide : Product  Inputs=*/
  Gain : Gain  Gain=2*pi
  Power : Math  Operator=pow
  Sqrt : Sqrt
  T : Outport
  wires:
  a/1 -> Power/1
  Constant/1 -> Power/2
  Power/1 -> Divide/1
  mu/1 -> Divide/2
  Divide/1 -> Sqrt/1
  Sqrt/1 -> Gain/1
  Gain/1 -> T/1

== system LIBRARY_SAD/Quaternion Omega matrix ==
  w_x : Inport
  w_y : Inport  Port=2
  w_z : Inport  Port=3
  0 : Inport  Port=4
  Gain{,1..5} (6 alike) : Gain  Gain=-1
  Vector Concatenate{,1..3} (4 alike) : Concatenate  NumInputs=4  Mode=Multidimensional array
  Vector Concatenate4 : Concatenate  NumInputs=4  Mode=Multidimensional array  ConcatenateDimension=2
  Omega Matrix : Outport
  wires:
  0/1 -> Vector Concatenate1/2, Vector Concatenate/1, Vector Concatenate2/3, Vector Concatenate3/4
  Gain1/1 -> Vector Concatenate/4
  Vector Concatenate1/1 -> Vector Concatenate4/2  "second column"
  Vector Concatenate2/1 -> Vector Concatenate4/3  "third column"
  w_z/1 -> Vector Concatenate1/1, Gain/1, Vector Concatenate3/3, Gain5/1
  w_y/1 -> Gain3/1, Gain4/1, Vector Concatenate3/2, Vector Concatenate/3
  Gain4/1 -> Vector Concatenate2/1
  Gain3/1 -> Vector Concatenate1/4
  Gain2/1 -> Vector Concatenate1/3
  Vector Concatenate3/1 -> Vector Concatenate4/4  "fourth column"
  Gain/1 -> Vector Concatenate/2
  Vector Concatenate/1 -> Vector Concatenate4/1  "first column"
  w_x/1 -> Gain1/1, Gain2/1, Vector Concatenate2/2, Vector Concatenate3/1
  Gain5/1 -> Vector Concatenate2/4
  Vector Concatenate4/1 -> Omega Matrix/1  "Omega Matrix"

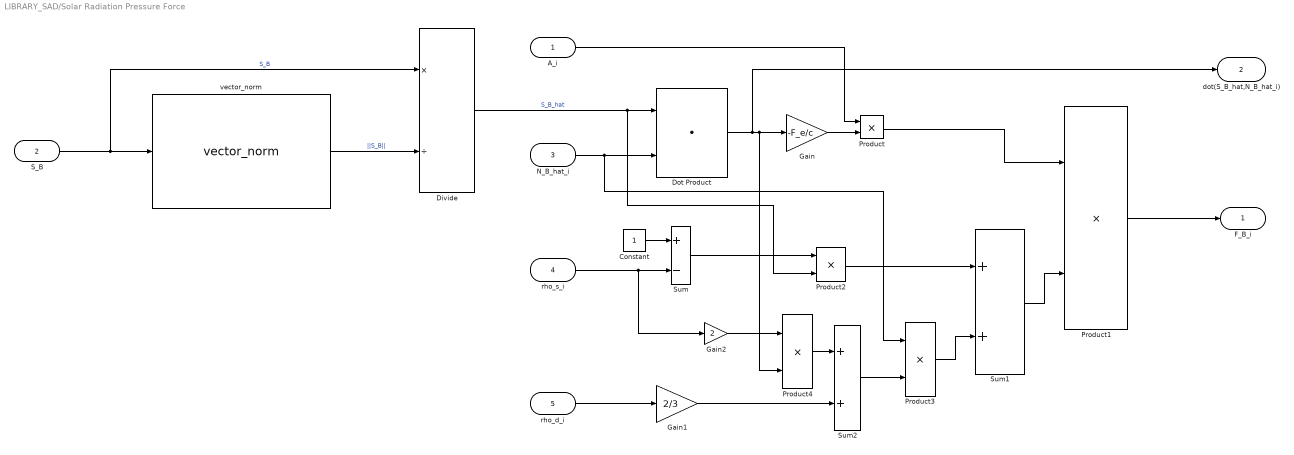
== system LIBRARY_SAD/Solar Radiation Pressure Force ==
  A_i : Inport
  S_B : Inport  Port=2
  N_B_hat_i : Inport  Port=3
  rho_s_i : Inport  Port=4
  rho_d_i : Inport  Port=5
  Constant : Constant
  Divide : Product  Inputs=*/
  Dot Product : DotProduct  OutDataTypeStr=Inherit: Inherit via internal rule
  Gain : Gain  Gain=-F_e/c
  Gain1 : Gain  Gain=2/3
  Gain2 : Gain  Gain=2
  Product{,1..4} (5 alike) : Product
  Sum : Sum  Inputs=+-
  Sum1 : Sum
  Sum2 : Sum
  vector_norm : $bdroot/vector_norm  SystemSampleTime=-1  VariantActivationTime=update diagram  EmptyChoice=off  PassThrough=off  PassThroughVariantControl=(default)  EmptyChoiceVariantControl=(default)  AllowFlexibleInterface=on  Latency=0  AutoFrameSizeCalculation=off
  F_B_i : Outport
  dot(S_B_hat,N_B_hat_i) : Outport  Port=2
  wires:
  Gain/1 -> Product/2
  A_i/1 -> Product/1
  N_B_hat_i/1 -> Product3/1, Dot Product/2
  Dot Product/1 -> dot(S_B_hat,N_B_hat_i)/1, Product4/2, Gain/1
  Product/1 -> Product1/1
  Constant/1 -> Sum/1
  rho_s_i/1 -> Gain2/1, Sum/2
  Sum/1 -> Product2/1
  Product2/1 -> Sum1/1
  Gain2/1 -> Product4/1
  Product4/1 -> Sum2/1
  rho_d_i/1 -> Gain1/1
  Gain1/1 -> Sum2/2
  Sum2/1 -> Product3/2
  Sum1/1 -> Product1/2
  Product1/1 -> F_B_i/1
  S_B/1 -> vector_norm/1, Divide/1  "S_B"
  Divide/1 -> Product2/2, Dot Product/1  "S_B_hat"
  vector_norm/1 -> Divide/2  "||S_B||"
  Product3/1 -> Sum1/2

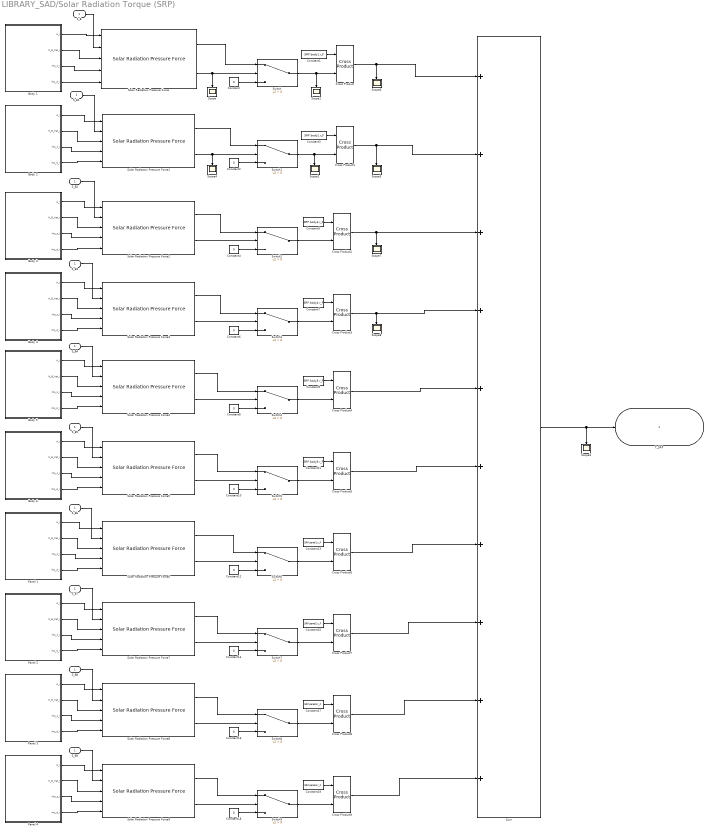
== system LIBRARY_SAD/Solar Radiation Torque (SRP) ==
  S_B : Inport
  Body 1 : Subsystem
  Body 2 : Subsystem
  Body 3 : Subsystem
  Body 4 : Subsystem
  Body 5 : Subsystem
  Body 6 : Subsystem
  Constant{,2,4,6,8,10,12,14,16,18} (10 alike) : Constant  Value=0
  Constant1 : Constant  Value=SRP.body1.r_F
  Constant11 : Constant  Value=SRP.body6.r_F
  Constant13 : Constant  Value=SRP.panel1.r_F
  Constant15 : Constant  Value=SRP.panel2.r_F
  Constant17 : Constant  Value=SRP.panel3.r_F
  Constant19 : Constant  Value=SRP.panel4.r_F
  Constant3 : Constant  Value=SRP.body2.r_F
  Constant5 : Constant  Value=SRP.body3.r_F
  Constant7 : Constant  Value=SRP.body4.r_F
  Constant9 : Constant  Value=SRP.body5.r_F
  Cross Product{,1..9} (10 alike) : matrix_library/Cross Product
  Panel 1 : Subsystem
  Panel 2 : Subsystem
  Panel 3 : Subsystem
  Panel 4 : Subsystem
  S_B{1..9} (9 alike) : InportShadow
  Scope{,1..8} (9 alike) : Scope
      Scope settings: ActiveDisplayYMinimum=-1  ActiveDisplayYMaximum=1  DataLoggingVariableName=ScopeData9
      Scope1 settings: ActiveDisplayYMinimum=-1  ActiveDisplayYMaximum=1  DataLoggingVariableName=ScopeData10
      Scope2 settings: ActiveDisplayYMinimum=-1  ActiveDisplayYMaximum=1  DataLoggingVariableName=ScopeData11
      Scope3 settings: ActiveDisplayYMinimum=-5.1359030627651383E-25  ActiveDisplayYMaximum=9.2718061255302776E-25  DataLoggingVariableName=ScopeData12
      Scope4 settings: ActiveDisplayYMinimum=-1  ActiveDisplayYMaximum=1  DataLoggingVariableName=ScopeData13
      Scope5 settings: ActiveDisplayYMinimum=-1  ActiveDisplayYMaximum=1  DataLoggingVariableName=ScopeData14
      Scope6 settings: ActiveDisplayYMinimum=-1  ActiveDisplayYMaximum=1  DataLoggingVariableName=ScopeData15
      Scope7 settings: ActiveDisplayYMinimum=-1  ActiveDisplayYMaximum=1  DataLoggingVariableName=ScopeData18
      Scope8 settings: ActiveDisplayYMinimum=-1  ActiveDisplayYMaximum=1  DataLoggingVariableName=ScopeData19
  Solar Radiation Pressure Force{,1..9} (10 alike) : lIBRARY_SAD_SAD/Solar Radiation Pressure Force  SystemSampleTime=-1  SSRTWFcnClass=[]  VariantActivationTime=update diagram  EmptyChoice=off  PassThrough=off  PassThroughVariantControl=(default)  EmptyChoiceVariantControl=(default)  AllowFlexibleInterface=on  Latency=0  AutoFrameSizeCalculation=off
  Sum : Sum  Inputs=++++++++++
  Switch{,1..9} (10 alike) : Switch  Criteria=u2 > Threshold  SaturateOnIntegerOverflow=off  InputSameDT=off
  T_SRP : Outport
  wires:
  S_B/1 -> Solar Radiation Pressure Force/2
  Body 1/1(A_i) -> Solar Radiation Pressure Force/1
  Body 1/2(N_B_hat_i) -> Solar Radiation Pressure Force/3
  Body 1/3(rho_s_i) -> Solar Radiation Pressure Force/4
  Body 1/4(rho_d_i) -> Solar Radiation Pressure Force/5
  Solar Radiation Pressure Force/1 -> Switch/1
  Solar Radiation Pressure Force/2 -> Scope/1, Switch/2
  Body 2/4(rho_d_i) -> Solar Radiation Pressure Force1/5
  Body 2/3(rho_s_i) -> Solar Radiation Pressure Force1/4
  Body 2/2(N_B_hat_i) -> Solar Radiation Pressure Force1/3
  Body 2/1(A_i) -> Solar Radiation Pressure Force1/1
  S_B1/1 -> Solar Radiation Pressure Force1/2
  S_B2/1 -> Solar Radiation Pressure Force2/2
  Body 3/1(A_i) -> Solar Radiation Pressure Force2/1
  Body 3/2(N_B_hat_i) -> Solar Radiation Pressure Force2/3
  Body 3/3(rho_s_i) -> Solar Radiation Pressure Force2/4
  Body 3/4(rho_d_i) -> Solar Radiation Pressure Force2/5
  Body 4/4(rho_d_i) -> Solar Radiation Pressure Force3/5
  Body 4/3(rho_s_i) -> Solar Radiation Pressure Force3/4
  Body 4/2(N_B_hat_i) -> Solar Radiation Pressure Force3/3
  Body 4/1(A_i) -> Solar Radiation Pressure Force3/1
  S_B3/1 -> Solar Radiation Pressure Force3/2
  S_B4/1 -> Solar Radiation Pressure Force4/2
  Body 5/1(A_i) -> Solar Radiation Pressure Force4/1
  Body 5/2(N_B_hat_i) -> Solar Radiation Pressure Force4/3
  Body 5/3(rho_s_i) -> Solar Radiation Pressure Force4/4
  Body 5/4(rho_d_i) -> Solar Radiation Pressure Force4/5
  Body 6/4(rho_d_i) -> Solar Radiation Pressure Force5/5
  Body 6/3(rho_s_i) -> Solar Radiation Pressure Force5/4
  Body 6/2(N_B_hat_i) -> Solar Radiation Pressure Force5/3
  Body 6/1(A_i) -> Solar Radiation Pressure Force5/1
  S_B5/1 -> Solar Radiation Pressure Force5/2
  S_B6/1 -> Solar Radiation Pressure Force6/2
  Panel 1/1(A_i) -> Solar Radiation Pressure Force6/1
  Panel 1/2(N_B_hat_i) -> Solar Radiation Pressure Force6/3
  Panel 1/3(rho_s_i) -> Solar Radiation Pressure Force6/4
  Panel 1/4(rho_d_i) -> Solar Radiation Pressure Force6/5
  Panel 2/4(rho_d_i) -> Solar Radiation Pressure Force7/5
  Panel 2/3(rho_s_i) -> Solar Radiation Pressure Force7/4
  Panel 2/2(N_B_hat_i) -> Solar Radiation Pressure Force7/3
  Panel 2/1(A_i) -> Solar Radiation Pressure Force7/1
  S_B7/1 -> Solar Radiation Pressure Force7/2
  S_B8/1 -> Solar Radiation Pressure Force8/2
  Panel 3/1(A_i) -> Solar Radiation Pressure Force8/1
  Panel 3/2(N_B_hat_i) -> Solar Radiation Pressure Force8/3
  Panel 3/3(rho_s_i) -> Solar Radiation Pressure Force8/4
  Panel 3/4(rho_d_i) -> Solar Radiation Pressure Force8/5
  Panel 4/4(rho_d_i) -> Solar Radiation Pressure Force9/5
  Panel 4/3(rho_s_i) -> Solar Radiation Pressure Force9/4
  Panel 4/2(N_B_hat_i) -> Solar Radiation Pressure Force9/3
  Panel 4/1(A_i) -> Solar Radiation Pressure Force9/1
  S_B9/1 -> Solar Radiation Pressure Force9/2
  Constant/1 -> Switch/3
  Switch/1 -> Scope1/1, Cross Product/2
  Constant1/1 -> Cross Product/1
  Cross Product/1 -> Scope6/1, Sum/1
  Cross Product1/1 -> Sum/2, Scope5/1
  Constant3/1 -> Cross Product1/1
  Switch1/1 -> Scope2/1, Cross Product1/2
  Constant2/1 -> Switch1/3
  Solar Radiation Pressure Force1/2 -> Scope4/1, Switch1/2
  Solar Radiation Pressure Force1/1 -> Switch1/1
  Solar Radiation Pressure Force2/1 -> Switch2/1
  Solar Radiation Pressure Force2/2 -> Switch2/2
  Constant4/1 -> Switch2/3
  Switch2/1 -> Cross Product2/2
  Constant5/1 -> Cross Product2/1
  Cross Product2/1 -> Scope7/1, Sum/3
  Cross Product3/1 -> Scope8/1, Sum/4
  Constant7/1 -> Cross Product3/1
  Switch3/1 -> Cross Product3/2
  Constant6/1 -> Switch3/3
  Solar Radiation Pressure Force3/2 -> Switch3/2
  Solar Radiation Pressure Force3/1 -> Switch3/1
  Solar Radiation Pressure Force4/1 -> Switch4/1
  Solar Radiation Pressure Force4/2 -> Switch4/2
  Constant8/1 -> Switch4/3
  Switch4/1 -> Cross Product4/2
  Constant9/1 -> Cross Product4/1
  Cross Product4/1 -> Sum/5
  Cross Product5/1 -> Sum/6
  Constant11/1 -> Cross Product5/1
  Switch5/1 -> Cross Product5/2
  Constant10/1 -> Switch5/3
  Solar Radiation Pressure Force5/2 -> Switch5/2
  Solar Radiation Pressure Force5/1 -> Switch5/1
  Solar Radiation Pressure Force6/1 -> Switch6/1
  Solar Radiation Pressure Force6/2 -> Switch6/2
  Constant12/1 -> Switch6/3
  Switch6/1 -> Cross Product6/2
  Constant13/1 -> Cross Product6/1
  Cross Product6/1 -> Sum/7
  Cross Product7/1 -> Sum/8
  Constant15/1 -> Cross Product7/1
  Switch7/1 -> Cross Product7/2
  Constant14/1 -> Switch7/3
  Solar Radiation Pressure Force7/2 -> Switch7/2
  Solar Radiation Pressure Force7/1 -> Switch7/1
  Solar Radiation Pressure Force8/1 -> Switch8/1
  Solar Radiation Pressure Force8/2 -> Switch8/2
  Constant16/1 -> Switch8/3
  Switch8/1 -> Cross Product8/2
  Constant17/1 -> Cross Product8/1
  Cross Product8/1 -> Sum/9
  Cross Product9/1 -> Sum/10
  Constant19/1 -> Cross Product9/1
  Switch9/1 -> Cross Product9/2
  Constant18/1 -> Switch9/3
  Solar Radiation Pressure Force9/2 -> Switch9/2
  Solar Radiation Pressure Force9/1 -> Switch9/1
  Sum/1 -> Scope3/1, T_SRP/1

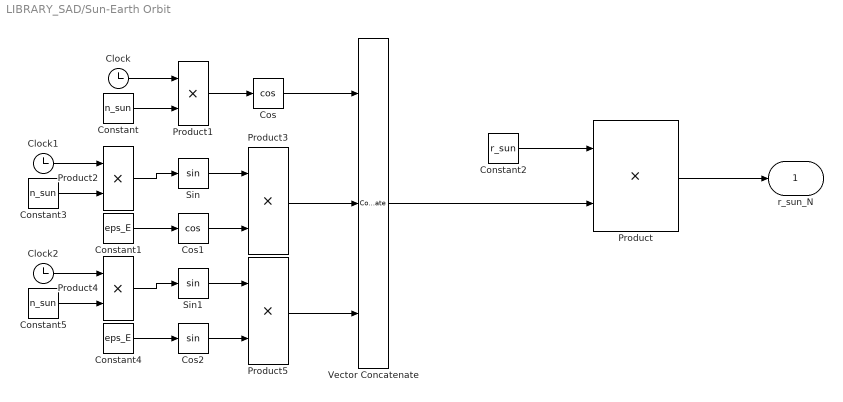
== system LIBRARY_SAD/Sun-Earth Orbit ==
  Clock : Clock
  Clock1 : Clock
  Clock2 : Clock
  Constant : Constant  Value=n_sun
  Constant1 : Constant  Value=eps_E
  Constant2 : Constant  Value=r_sun
  Constant3 : Constant  Value=n_sun
  Constant4 : Constant  Value=eps_E
  Constant5 : Constant  Value=n_sun
  Cos : Trigonometry  Operator=cos
  Cos1 : Trigonometry  Operator=cos
  Cos2 : Trigonometry
  Product{,1..5} (6 alike) : Product
  Sin : Trigonometry
  Sin1 : Trigonometry
  Vector Concatenate : Concatenate  NumInputs=3
  r_sun_N : Outport
  wires:
  Constant2/1 -> Product/1
  Clock/1 -> Product1/1
  Constant/1 -> Product1/2
  Product1/1 -> Cos/1
  Cos/1 -> Vector Concatenate/1
  Product2/1 -> Sin/1
  Constant3/1 -> Product2/2
  Clock1/1 -> Product2/1
  Sin/1 -> Product3/1
  Constant1/1 -> Cos1/1
  Product3/1 -> Vector Concatenate/2
  Cos1/1 -> Product3/2
  Cos2/1 -> Product5/2
  Product5/1 -> Vector Concatenate/3
  Constant4/1 -> Cos2/1
  Sin1/1 -> Product5/1
  Clock2/1 -> Product4/1
  Constant5/1 -> Product4/2
  Product4/1 -> Sin1/1
  Vector Concatenate/1 -> Product/2
  Product/1 -> r_sun_N/1

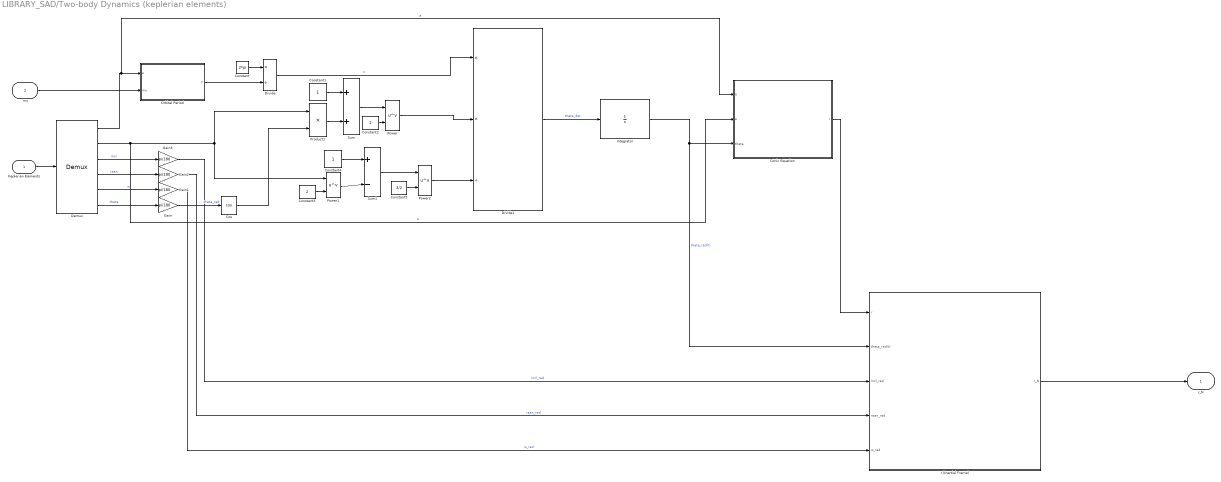
== system LIBRARY_SAD/Two-body Dynamics (keplerian elements) ==
  Keplerian Elements : Inport
  mu : Inport  Port=2
  Conic Equation : Subsystem
  Constant : Constant  Value=2*pi
  Constant1 : Constant
  Constant2 : Constant  Value=2
  Constant3 : Constant  Value=2
  Constant4 : Constant
  Constant5 : Constant  Value=3/2
  Cos : Trigonometry  Operator=cos
  Demux : Demux  Outputs=6
      settings: DisplayOption=none
  Divide : Product  Inputs=*/
  Divide1 : Product  Inputs=**/
  Gain{,1..3} (4 alike) : Gain  Gain=pi/180
  Integrator : Integrator  InitialCondition=theta*(pi/180)  WrapState=on  WrappedStateUpperValue=2*pi  WrappedStateLowerValue=0
  Orbital Period : Subsystem
  Power : Math  Operator=pow
  Power1 : Math  Operator=pow
  Power2 : Math  Operator=pow
  Product1 : Product
  Sum : Sum
  Sum1 : Sum  Inputs=+-
  r (Inertial Frame) : Subsystem
  r_N : Outport
  wires:
  Keplerian Elements/1 -> Demux/1
  Demux/1 -> Conic Equation/1(a), Orbital Period/1(a)  "a"
  Demux/2 -> Conic Equation/2(e), Product1/1, Power1/1  "e"
  Demux/3 -> Gain3/1  "incl"
  Demux/4 -> Gain2/1  "raan"
  Demux/5 -> Gain1/1  "w"
  Demux/6 -> Gain/1  "theta"
  mu/1 -> Orbital Period/2(mu)
  Orbital Period/1(T) -> Divide/2
  Constant/1 -> Divide/1
  Divide/1 -> Divide1/1  "n"
  Gain/1 -> Cos/1  "theta_rad"
  Constant1/1 -> Sum/1
  Cos/1 -> Product1/2
  Product1/1 -> Sum/2
  Sum/1 -> Power/1
  Constant2/1 -> Power/2
  Power/1 -> Divide1/2
  Constant3/1 -> Power1/2
  Power1/1 -> Sum1/2
  Constant4/1 -> Sum1/1
  Constant5/1 -> Power2/2
  Sum1/1 -> Power2/1
  Power2/1 -> Divide1/3
  Divide1/1 -> Integrator/1  "theta_dot"
  Integrator/1 -> r (Inertial Frame)/2(theta_rad(t)), Conic Equation/3(theta)  "theta_rad(t)"
  Conic Equation/1(r) -> r (Inertial Frame)/1(r)
  Gain3/1 -> r (Inertial Frame)/3(incl_rad)  "incl_rad"
  Gain2/1 -> r (Inertial Frame)/4(raan_rad)  "raan_rad"
  Gain1/1 -> r (Inertial Frame)/5(w_rad)  "w_rad"
  r (Inertial Frame)/1(r_N) -> r_N/1

== system LIBRARY_SAD/vector_norm ==
  r : Inport
  Sqrt : Sqrt
  Square : Math  Operator=square
  Sum of Elements : Sum  Inputs=+
  r_norm : Outport
  wires:
  Square/1 -> Sum of Elements/1
  Sum of Elements/1 -> Sqrt/1
  r/1 -> Square/1
  Sqrt/1 -> r_norm/1

== system LIBRARY_SAD/Earth-S//C Orbit/Conic Equation ==
  a : Inport
  e : Inport  Port=2
  theta_rad(t) : Inport  Port=3
  Constant : Constant  Value=2
  Constant1 : Constant
  Constant2 : Constant
  Cos : Trigonometry  Operator=cos
  Divide : Product  Inputs=*/
  Power : Math  Operator=pow
  Product : Product
  Product1 : Product
  Sum : Sum  Inputs=+-
  Sum1 : Sum
  r : Outport
  wires:
  a/1 -> Product/1
  e/1 -> Product1/1, Power/1
  Constant/1 -> Power/2
  Power/1 -> Sum/2
  Constant1/1 -> Sum/1
  Sum/1 -> Product/2
  Product/1 -> Divide/1
  Divide/1 -> r/1
  Constant2/1 -> Sum1/1
  theta_rad(t)/1 -> Cos/1
  Cos/1 -> Product1/2
  Product1/1 -> Sum1/2
  Sum1/1 -> Divide/2

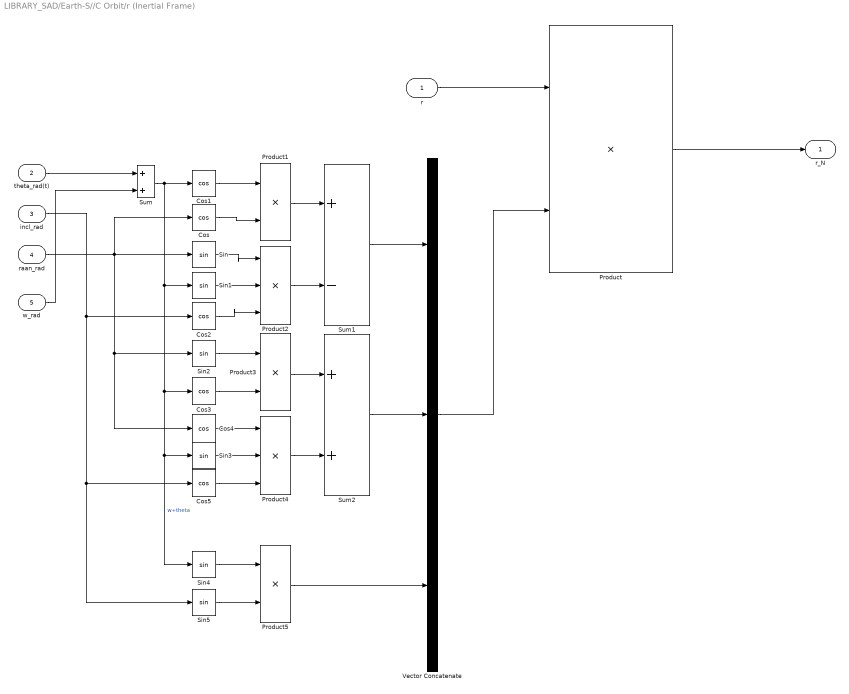
== system LIBRARY_SAD/Earth-S//C Orbit/r (Inertial Frame) ==
  r : Inport
  theta_rad(t) : Inport  Port=2
  incl_rad : Inport  Port=3
  raan_rad : Inport  Port=4
  w_rad : Inport  Port=5
  Cos{,1..5} (6 alike) : Trigonometry  Operator=cos
  Product{,1,3,5} (4 alike) : Product
  Product2 : Product  Inputs=3
  Product4 : Product  Inputs=3
  Sin{,1..5} (6 alike) : Trigonometry
  Sum : Sum
  Sum1 : Sum  Inputs=+-
  Sum2 : Sum
  Vector Concatenate : Concatenate  NumInputs=3
  r_N : Outport
  wires:
  r/1 -> Product/1
  raan_rad/1 -> Cos/1, Cos4/1, Sin2/1, Sin/1
  w_rad/1 -> Sum/2
  Cos/1 -> Product1/2
  theta_rad(t)/1 -> Sum/1
  Sum/1 -> Sin4/1, Sin3/1, Cos3/1, Sin1/1, Cos1/1  "w+theta"
  Cos1/1 -> Product1/1
  Product1/1 -> Sum1/1
  Product2/1 -> Sum1/2
  Sin/1 -> Product2/1
  Sin1/1 -> Product2/2
  Cos2/1 -> Product2/3
  incl_rad/1 -> Cos5/1, Sin5/1, Cos2/1
  Sum1/1 -> Vector Concatenate/1
  Sum2/1 -> Vector Concatenate/2
  Sin2/1 -> Product3/1
  Cos3/1 -> Product3/2
  Product3/1 -> Sum2/1
  Product4/1 -> Sum2/2
  Cos4/1 -> Product4/1
  Sin3/1 -> Product4/2
  Cos5/1 -> Product4/3
  Sin4/1 -> Product5/1
  Sin5/1 -> Product5/2
  Product5/1 -> Vector Concatenate/3
  Vector Concatenate/1 -> Product/2
  Product/1 -> r_N/1

== system LIBRARY_SAD/Euler Equations (scalar, torque-free)/w_x_dot ==
  w_y : Inport
  w_z : Inport  Port=2
  Constant : Constant  Value=Iy
  Constant1 : Constant  Value=Iz
  Constant2 : Constant  Value=Ix
  Divide : Product  Inputs=**/
  Product : Product
  Sum : Sum  Inputs=+-
  w_x_dot : Outport
  wires:
  Constant2/1 -> Divide/3
  Sum/1 -> Divide/2
  Divide/1 -> w_x_dot/1
  Constant1/1 -> Sum/2
  Constant/1 -> Sum/1
  Product/1 -> Divide/1
  w_z/1 -> Product/2
  w_y/1 -> Product/1

== system LIBRARY_SAD/Euler Equations (scalar, torque-free)/w_y_dot ==
  w_x : Inport
  w_z : Inport  Port=2
  Constant : Constant  Value=Iz
  Constant1 : Constant  Value=Ix
  Constant2 : Constant  Value=Iy
  Divide : Product  Inputs=**/
  Product : Product
  Sum : Sum  Inputs=+-
  w_y_dot : Outport
  wires:
  Constant2/1 -> Divide/3
  Constant1/1 -> Sum/2
  Constant/1 -> Sum/1
  Sum/1 -> Divide/2
  w_z/1 -> Product/2
  Divide/1 -> w_y_dot/1
  w_x/1 -> Product/1
  Product/1 -> Divide/1

== system LIBRARY_SAD/Euler Equations (scalar, torque-free)/w_z_dot ==
  w_x : Inport
  w_y : Inport  Port=2
  Constant : Constant  Value=Ix
  Constant1 : Constant  Value=Iy
  Constant2 : Constant  Value=Iz
  Divide : Product  Inputs=**/
  Product : Product
  Sum : Sum  Inputs=+-
  w_z_dot : Outport
  wires:
  Product/1 -> Divide/1
  w_x/1 -> Product/1
  Divide/1 -> w_z_dot/1
  w_y/1 -> Product/2
  Sum/1 -> Divide/2
  Constant/1 -> Sum/1
  Constant1/1 -> Sum/2
  Constant2/1 -> Divide/3

== system LIBRARY_SAD/Magnetic Torque (Simple Dipole Model) /B_N (Simple Dipole Model) ==
  r_S/C_N : Inport
  Clock : Clock
  Constant : Constant  Value=Re
  Constant1 : Constant  Value=3
  Constant2 : Constant  Value=3
  Divide : Product  Inputs=*/
  Divide1 : Product  Inputs=***/
  Dot Product : DotProduct  OutDataTypeStr=Inherit: Inherit via internal rule
  Earth's Magnetic Dipole (unit vector) : Subsystem
  Gain : Gain  Gain=3
  H_0 : Subsystem
  Power : Math  Operator=pow
  Power1 : Math  Operator=pow
  Product : Product
  Subtract : Sum  Inputs=+-
  vector_norm : lIBRARY_SAD_SAD/vector_norm  SystemSampleTime=-1  SSRTWFcnClass=[]  VariantActivationTime=update diagram  EmptyChoice=off  PassThrough=off  PassThroughVariantControl=(default)  EmptyChoiceVariantControl=(default)  AllowFlexibleInterface=on  Latency=0  AutoFrameSizeCalculation=off
  B_N : Outport
  wires:
  Clock/1 -> Earth's Magnetic Dipole (unit vector)/1(Time)
  Constant/1 -> Power/1
  Product/1 -> Subtract/1
  Divide/1 -> Dot Product/1, Product/1  "r_hat"
  Constant1/1 -> Power/2
  Divide1/1 -> B_N/1
  Subtract/1 -> Divide1/1
  Power/1 -> Divide1/2
  Power1/1 -> Divide1/4
  H_0/1(H_0) -> Divide1/3
  Dot Product/1 -> Gain/1
  Constant2/1 -> Power1/2
  vector_norm/1 -> Divide/2, Power1/1  "||r_S/C_N||"
  r_S/C_N/1 -> Divide/1, vector_norm/1
  Gain/1 -> Product/2
  Earth's Magnetic Dipole (unit vector)/1(m_hat) -> Subtract/2, Dot Product/2  "m_hat"

== system LIBRARY_SAD/Solar Radiation Torque (SRP)/Body 1 ==
  Constant : Constant  Value=SRP.body1.A
  Constant1 : Constant  Value=SRP.body1.N_hat
  Constant2 : Constant  Value=SRP.body1.rho_s
  Constant3 : Constant  Value=SRP.body1.rho_d
  A_i : Outport
  N_B_hat_i : Outport  Port=2
  rho_s_i : Outport  Port=3
  rho_d_i : Outport  Port=4
  wires:
  Constant/1 -> A_i/1
  Constant1/1 -> N_B_hat_i/1
  Constant2/1 -> rho_s_i/1
  Constant3/1 -> rho_d_i/1

== system LIBRARY_SAD/Solar Radiation Torque (SRP)/Body 2 ==
  Constant : Constant  Value=SRP.body2.A
  Constant1 : Constant  Value=SRP.body2.N_hat
  Constant2 : Constant  Value=SRP.body2.rho_s
  Constant3 : Constant  Value=SRP.body2.rho_d
  A_i : Outport
  N_B_hat_i : Outport  Port=2
  rho_s_i : Outport  Port=3
  rho_d_i : Outport  Port=4
  wires:
  Constant3/1 -> rho_d_i/1
  Constant2/1 -> rho_s_i/1
  Constant1/1 -> N_B_hat_i/1
  Constant/1 -> A_i/1

== system LIBRARY_SAD/Solar Radiation Torque (SRP)/Body 3 ==
  Constant : Constant  Value=SRP.body3.A
  Constant1 : Constant  Value=SRP.body3.N_hat
  Constant2 : Constant  Value=SRP.body3.rho_s
  Constant3 : Constant  Value=SRP.body3.rho_d
  A_i : Outport
  N_B_hat_i : Outport  Port=2
  rho_s_i : Outport  Port=3
  rho_d_i : Outport  Port=4
  wires:
  Constant/1 -> A_i/1
  Constant1/1 -> N_B_hat_i/1
  Constant2/1 -> rho_s_i/1
  Constant3/1 -> rho_d_i/1

== system LIBRARY_SAD/Solar Radiation Torque (SRP)/Body 4 ==
  Constant : Constant  Value=SRP.body4.A
  Constant1 : Constant  Value=SRP.body4.N_hat
  Constant2 : Constant  Value=SRP.body4.rho_s
  Constant3 : Constant  Value=SRP.body4.rho_d
  A_i : Outport
  N_B_hat_i : Outport  Port=2
  rho_s_i : Outport  Port=3
  rho_d_i : Outport  Port=4
  wires:
  Constant3/1 -> rho_d_i/1
  Constant2/1 -> rho_s_i/1
  Constant1/1 -> N_B_hat_i/1
  Constant/1 -> A_i/1

== system LIBRARY_SAD/Solar Radiation Torque (SRP)/Body 5 ==
  Constant : Constant  Value=SRP.body5.A
  Constant1 : Constant  Value=SRP.body5.N_hat
  Constant2 : Constant  Value=SRP.body5.rho_s
  Constant3 : Constant  Value=SRP.body5.rho_d
  A_i : Outport
  N_B_hat_i : Outport  Port=2
  rho_s_i : Outport  Port=3
  rho_d_i : Outport  Port=4
  wires:
  Constant/1 -> A_i/1
  Constant1/1 -> N_B_hat_i/1
  Constant2/1 -> rho_s_i/1
  Constant3/1 -> rho_d_i/1

== system LIBRARY_SAD/Solar Radiation Torque (SRP)/Body 6 ==
  Constant : Constant  Value=SRP.body6.A
  Constant1 : Constant  Value=SRP.body6.N_hat
  Constant2 : Constant  Value=SRP.body6.rho_s
  Constant3 : Constant  Value=SRP.body6.rho_d
  A_i : Outport
  N_B_hat_i : Outport  Port=2
  rho_s_i : Outport  Port=3
  rho_d_i : Outport  Port=4
  wires:
  Constant3/1 -> rho_d_i/1
  Constant2/1 -> rho_s_i/1
  Constant1/1 -> N_B_hat_i/1
  Constant/1 -> A_i/1

== system LIBRARY_SAD/Solar Radiation Torque (SRP)/Panel 1 ==
  Constant : Constant  Value=SRP.panel1.A
  Constant1 : Constant  Value=SRP.panel1.N_hat
  Constant2 : Constant  Value=SRP.panel1.rho_s
  Constant3 : Constant  Value=SRP.panel1.rho_d
  A_i : Outport
  N_B_hat_i : Outport  Port=2
  rho_s_i : Outport  Port=3
  rho_d_i : Outport  Port=4
  wires:
  Constant/1 -> A_i/1
  Constant1/1 -> N_B_hat_i/1
  Constant2/1 -> rho_s_i/1
  Constant3/1 -> rho_d_i/1

== system LIBRARY_SAD/Solar Radiation Torque (SRP)/Panel 2 ==
  Constant : Constant  Value=SRP.panel2.A
  Constant1 : Constant  Value=SRP.panel2.N_hat
  Constant2 : Constant  Value=SRP.panel2.rho_s
  Constant3 : Constant  Value=SRP.panel2.rho_d
  A_i : Outport
  N_B_hat_i : Outport  Port=2
  rho_s_i : Outport  Port=3
  rho_d_i : Outport  Port=4
  wires:
  Constant3/1 -> rho_d_i/1
  Constant2/1 -> rho_s_i/1
  Constant1/1 -> N_B_hat_i/1
  Constant/1 -> A_i/1
